simulink model "Parent"  (R2023a)
settings: Solver=FixedStepAuto  StartTime=0.0  StopTime=inf  RelTol=1e-3
undefined symbols (not defined in the file): map
libraries: androidcommunicationlib x5, androiduilib x5, androidaudiovideolib x3
settings Model: Creator=tamiz  LastModifiedBy=tamiz
settings OptimizationCC: EnhancedBackFolding=on  PassReuseOutputArgsAs=Individual arguments  ZeroExternalMemoryAtStartup=off  ZeroInternalMemoryAtStartup=off  MaxStackSize=64  OptimizeBlockOrder=speed  DifferentSizesBufferReuse=on  OptimizationCustomize=off  EfficientTunableParamExpr=on
settings DebuggingCC: ParameterTunabilityLossMsg=error
settings HardwareCC: ProdBitPerPointer=32  ProdBitPerSizeT=32  ProdBitPerPtrDiffT=32  ProdLargestAtomicInteger=Long  ProdLargestAtomicFloat=Double  ProdWordSize=32  ProdHWDeviceType=ARM Compatible->ARM Cortex
settings SFSimCC: MATLABDynamicMemAlloc=off
settings RTWCC: Description=Embedded Coder  SystemTargetFile=ert.tlc  HardwareBoard=Android Device  TLCOptions="-aInlineSetEventsForThisBaseRateFcn=TLC_FALSE -aSuppressMultiTaskScheduler=TLC_FALSE  -aRateBasedStepFcn=0"  TemplateMakefile=ert_default_tmf  RTWVerbose=off  Toolchain=Android SDK/NDK Tools
settings CodeAppCC: ForceParamTrailComments=on  IgnoreCustomStorageClasses=off  OperatorAnnotations=on  SimulinkDataObjDesc=on  SFDataObjDesc=on  InsertBlockDesc=on

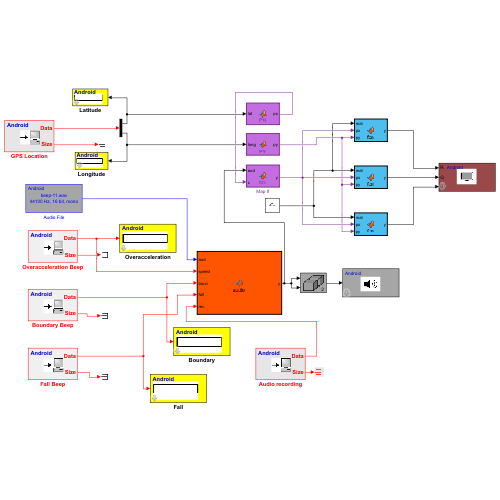
[thumbnail: Simulink's stored preview of the top-level diagram]
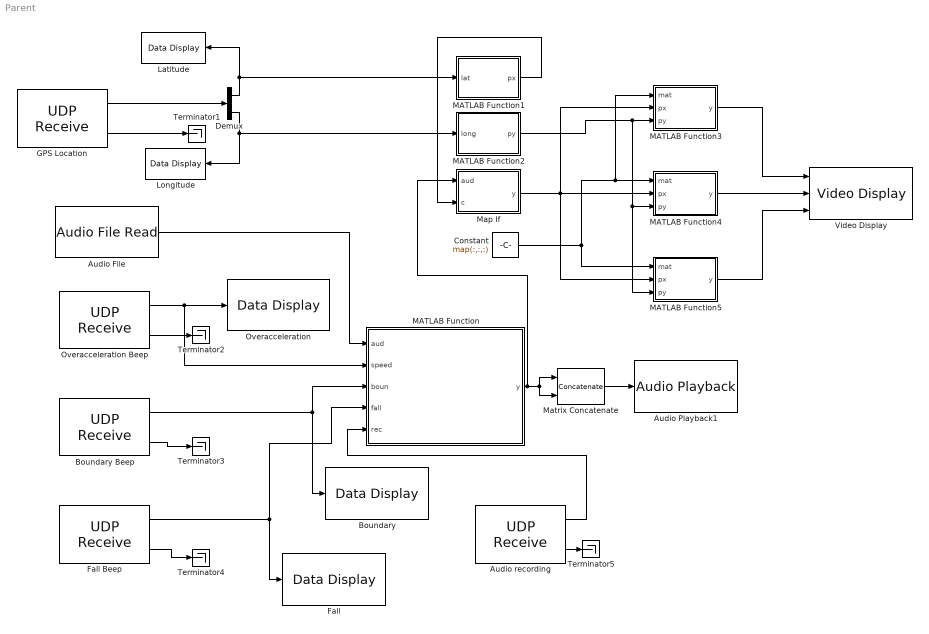
== system Parent ==
  Audio File : androidaudiovideolib/Audio File Read  FileName=C:\Users\tamiz\Downloads\beep-11.wav  FrameSize=4410
  Audio Playback1 : androidaudiovideolib/Audio Playback  SampleFreq=44100  AudioSamplingFreq=44100  SampleTime=0.1  DeviceStr=0  QueueDuration=0  BlockPlatform=Android
  Audio recording : androidcommunicationlib/UDP Receive  localURL='0.0.0.0'  localPort=25004  remoteURL='0.0.0.0'  remotePort=-1  recvBufferSize=8192  signalDatatype=int16  dims=4410  isVarSize=off  showBlockingTime=off  blockingTime=0  sampletime=0.1  blockPlatform=Android
  Boundary : androiduilib/Data Display  DataDisplayId=Parent/Boundary  Format=Integer  Precision=6  SimulateUsing=Code generation  blockPlatform=Android
  Boundary Beep : androidcommunicationlib/UDP Receive  localURL='0.0.0.0'  localPort=25002  remoteURL='0.0.0.0'  remotePort=-1  recvBufferSize=8192  signalDatatype=boolean  dims=1  isVarSize=off  showBlockingTime=off  blockingTime=0  sampletime=0.1  blockPlatform=Android
  Constant : Constant  Value=map(:,:,:)  VectorParams1D=off  SampleTime=0.1
  Demux : Demux  Outputs=2
  Fall : androiduilib/Data Display  DataDisplayId=Parent/Fall  Format=Integer  Precision=6  SimulateUsing=Code generation  blockPlatform=Android
  Fall Beep : androidcommunicationlib/UDP Receive  localURL='0.0.0.0'  localPort=25001  remoteURL='0.0.0.0'  remotePort=-1  recvBufferSize=8192  signalDatatype=boolean  dims=1  isVarSize=off  showBlockingTime=off  blockingTime=0  sampletime=0.1  blockPlatform=Android
  GPS Location : androidcommunicationlib/UDP Receive  localURL='0.0.0.0'  localPort=25000  remoteURL='0.0.0.0'  remotePort=-1  recvBufferSize=8192  signalDatatype=double  dims=2  isVarSize=off  showBlockingTime=off  blockingTime=0  sampletime=0.1  blockPlatform=Android
  Latitude : androiduilib/Data Display  DataDisplayId=Parent/Latitude  Format=Float  Precision=10  SimulateUsing=Code generation  blockPlatform=Android
  Longitude : androiduilib/Data Display  DataDisplayId=Parent/Longitude  Format=Float  Precision=10  SimulateUsing=Code generation  blockPlatform=Android
  MATLAB Function : MATLAB Function  TreatAsAtomicUnit=on
  MATLAB Function1 : MATLAB Function  TreatAsAtomicUnit=on
  MATLAB Function2 : MATLAB Function  TreatAsAtomicUnit=on
  MATLAB Function3 : MATLAB Function  TreatAsAtomicUnit=on
  MATLAB Function4 : MATLAB Function  TreatAsAtomicUnit=on
  MATLAB Function5 : MATLAB Function  TreatAsAtomicUnit=on
  Map If : MATLAB Function  TreatAsAtomicUnit=on
  Matrix Concatenate : Concatenate  Mode=Multidimensional array  ConcatenateDimension=2
  Overacceleration : androiduilib/Data Display  DataDisplayId=Parent/Overacceleration  Format=Integer  Precision=6  SimulateUsing=Code generation  blockPlatform=Android
  Overacceleration Beep : androidcommunicationlib/UDP Receive  localURL='0.0.0.0'  localPort=25003  remoteURL='0.0.0.0'  remotePort=-1  recvBufferSize=8192  signalDatatype=boolean  dims=1  isVarSize=off  showBlockingTime=off  blockingTime=0  sampletime=0.1  blockPlatform=Android
  Terminator{1..5} (5 alike) : Terminator
  Video Display : androidaudiovideolib/Video Display  BlockPlatform=Android
  wires:
  GPS Location/2 -> Terminator1/1
  GPS Location/1 -> Demux/1
  Demux/1 -> Latitude/1, MATLAB Function1/1(lat)
  Demux/2 -> Longitude/1, MATLAB Function2/1(long)
  Overacceleration Beep/2 -> Terminator2/1
  Boundary Beep/2 -> Terminator3/1
  Fall Beep/2 -> Terminator4/1
  Overacceleration Beep/1 -> Overacceleration/1, MATLAB Function/2(speed)
  Boundary Beep/1 -> MATLAB Function/3(boun), Boundary/1
  Fall Beep/1 -> MATLAB Function/4(fall), Fall/1
  Audio recording/2 -> Terminator5/1
  Audio recording/1 -> MATLAB Function/5(rec)
  Audio File/1 -> MATLAB Function/1(aud)
  Matrix Concatenate/1 -> Audio Playback1/1
  MATLAB Function/1(y) -> Map If/1(aud), Matrix Concatenate/2, Matrix Concatenate/1
  MATLAB Function2/1(py) -> MATLAB Function4/3(py), MATLAB Function5/3(py), MATLAB Function3/3(py)
  MATLAB Function3/1(y) -> Video Display/1
  MATLAB Function4/1(y) -> Video Display/2
  MATLAB Function5/1(y) -> Video Display/3
  Constant/1 -> MATLAB Function3/1(mat), MATLAB Function4/1(mat), MATLAB Function5/1(mat)
  MATLAB Function1/1(px) -> Map If/2(c)
  Map If/1(y) -> MATLAB Function3/2(px), MATLAB Function5/2(px), MATLAB Function4/2(px)

== matlab function Parent/MATLAB Function1 ==
  data: lat input; px output
function px = PX(lat)
    x = 352 - ((23.211137 - lat)* 352/0.001721);
    px = int16(x);
end

== matlab function Parent/MATLAB Function ==
  data: aud input; y output; speed input; boun input; fall input; rec input
function y = audio(aud, speed, boun, fall, rec)
    persistent micOn;
    if isempty(micOn)
        micOn = false;
    end
    
    if (fall == false)
        micOn = false;
    end 
    
    if (fall == true)
        y = aud;
        
        if rec ~= zeros(4410,1,'int16')
            micOn = true;
        end

        if micOn == true
            y = rec;
        end
    elseif (speed == true) || (boun == true)
        y = aud;
    else
        y = zeros(4410,1,'int16');
    end
end

== matlab function Parent/MATLAB Function2 ==
  data: long input; py output
function py = PY(long)
    y = 412 - ((72.682927 - long)* 412/0.002205);
    py = int16(y);
end

== matlab function Parent/MATLAB Function3 ==
  data: mat input; y output; px input; py input
function y = fcn(mat,px,py)
    px = max(10, min(px, size(mat, 1) - 10));
    py = max(10, min(py, size(mat, 2) - 10));
    y = mat(:, :, 1);
    y(px - 10:px + 10, py - 10:py + 10) = 255;
end

== matlab function Parent/MATLAB Function4 ==
  data: mat input; y output; px input; py input
function y = fcn(mat,px,py)
    px = max(10, min(px, size(mat, 1) - 10));
    py = max(10, min(py, size(mat, 2) - 10));
    y = mat(:, :, 2);
    y(px - 10:px + 10, py - 10:py + 10) = 0;
end

== matlab function Parent/MATLAB Function5 ==
  data: mat input; y output; px input; py input
function y = fcn(mat,px,py)
    px = max(10, min(px, size(mat, 1) - 10));
    py = max(10, min(py, size(mat, 2) - 10));
    y = mat(:, :, 3);
    y(px - 10:px + 10, py - 10:py + 10) = 0;
end

== matlab function Parent/Map If ==
  data: aud input; y output; c input
function y = fcn(aud,c)
    if aud ~= zeros(4410,1,'int16')
        y = c;
    else
        y = int16(1599);
    end
end
